simulink model "nonlinsim"  (R2020a)
settings: Solver=VariableStepAuto  StartTime=0.0  StopTime=10.0  RelTol=1e-3
values from neighbouring files (symbols this model uses):
  g = p(6)    [NLS_Dynamics.m]    (also in Project_Problem3.m = 3.711; linsim_script.m = 3.711; nonlinsim_script.m = 3.711)
  Gain = 93298    [linsim_script.m]    (also in nonlinsim_script.m)
  Kd = 9000    [Project_Problem5.m]    (also in linsim_script.m; nonlinsim_script.m = 60000)
  Ki = 1    [Project_Problem5.m]    (also in linsim_script.m = 0.5; nonlinsim_script.m = 200)
  Kp = 5000    [Project_Problem5.m]    (also in linsim_script.m; nonlinsim_script.m = 30000)
  M = p(1)    [NLS_Dynamics.m]    (also in Project_Problem3.m = 1025; linsim_script.m = 1025; nonlinsim_script.m = 1025)
  m = p(2)    [NLS_Dynamics.m]    (also in Project_Problem3.m = 500; linsim_script.m = 500; nonlinsim_script.m = 500)
  Poles = [-0.0008+1.0000i -0.0008-1.0000i -10.23]    [linsim_script.m]    (also in nonlinsim_script.m)
  r1o = 0    [nonlinsim_script.m]
  r2o = 0    [nonlinsim_script.m]
  u1o = (M+m)*g    (= 5659.275)    [nonlinsim_script.m]
  u2o = 0    [nonlinsim_script.m]
  u3o = 0    [nonlinsim_script.m]
  Zeros = [-0.3126 -0.5807 -0.8273]    [linsim_script.m]    (also in nonlinsim_script.m)
libraries: simulink x3
settings Model: Creator=zuzan  LastModifiedBy=zuzan

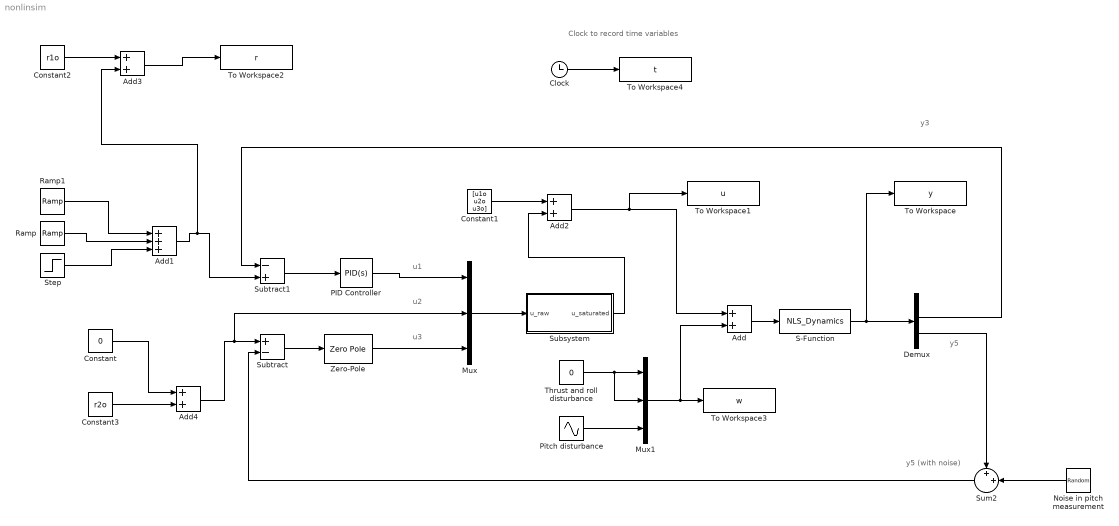
== system nonlinsim ==
  note: y5
  note: u1
  note: y5 (with noise)
  note: u2
  note: Clock to record time variables
  note: y3
  note: u3
  Add{,2..4} (4 alike) : Sum
  Add1 : Sum  Inputs=+++
  Clock : Clock
  Constant : Constant  Value=0
  Constant1 : Constant  Value=[u1o u2o u3o]
  Constant2 : Constant  Value=r1o
  Constant3 : Constant  Value=r2o
  Demux : Demux  Outputs=6
  Mux : Mux  Inputs=3
  Mux1 : Mux  Inputs=3
  Noise in pitch measurement : RandomNumber  Variance=1e-3  SampleTime=0.01
  PID Controller : simulink/Continuous/PID Controller  Controller=PID  Form=Parallel  TimeDomain=Continuous-time  UseExternalTs=off  SampleTime=-1  IntegratorMethod=Forward Euler  FilterMethod=Forward Euler  ControllerParametersSource=internal  P=Kp  I=Ki  D=Kd  UseFilter=on  N=100  TunerSelectOption=Transfer Function Based (PID Tuner App)  InitialConditionSource=internal  InitialConditionForIntegrator=0  InitialConditionForFilter=0  DifferentiatorICPrevScaledInput=0  ExternalReset=none  TrackingMode=off  Kt=1  LimitOutput=off  UpperSaturationLimit=inf  LowerSaturationLimit=-inf  LinearizeAsGain=on  AntiWindupMode=none  Kb=1  POutMin=[]  POutMax=[]  IOutMin=[]  IOutMax=[]  DOutMin=[]  DOutMax=[]  NOutMin=[]  NOutMax=[]  SumOutMin=[]  SumOutMax=[]  SaturationOutMin=[]  SaturationOutMax=[]  PParamMin=[]  PParamMax=[]  IParamMin=[]  IParamMax=[]  DParamMin=[]  DParamMax=[]  NParamMin=[]  NParamMax=[]  KbParamMin=[]  KbParamMax=[]  KtParamMin=[]  KtParamMax=[]  KbOutMin=[]  KbOutMax=[]  KtOutMin=[]  KtOutMax=[]  IntegratorOutMin=[]  IntegratorOutMax=[]  FilterOutMin=[]  FilterOutMax=[]  SumI1OutMin=[]  SumI1OutMax=[]  SumI2OutMin=[]  SumI2OutMax=[]  SumI3OutMin=[]  SumI3OutMax=[]  SumI4OutMin=[]  SumI4OutMax=[]  SumDOutMin=[]  SumDOutMax=[]  DifferentiatorOutMin=[]  DifferentiatorOutMax=[]  FilterDiffOutCoefMin=[]  FilterDiffOutCoefMax=[]  ReciprocalOutMin=[]  ReciprocalOutMax=[]  SumDenOutMin=[]  SumDenOutMax=[]  SumNumOutMin=[]  SumNumOutMax=[]  DivideOutMin=[]  DivideOutMax=[]  UdiffTsProdOutMin=[]  UdiffTsProdOutMax=[]  NTsProdOutMin=[]  NTsProdOutMax=[]  UintegralTsProdOutMin=[]  UintegralTsProdOutMax=[]  UngainTsProdOutMin=[]  UngainTsProdOutMax=[]  IntegratorContinuousStateAttributes=''  IntegratorStateMustResolveToSignalObject=off  IntegratorRTWStateStorageClass=Auto  FilterContinuousStateAttributes=''  FilterStateMustResolveToSignalObject=off  FilterRTWStateStorageClass=Auto  ParallelPVariant=InternalParameters  IdealPVariant=Disabled  IVariant=InternalParameters  DVariant=InternalParameters  IntegratorVariant=Continuous  SatVariant=Disabled  AWVariant=Passthrough  PCopyVariant=Disabled  TRVariant=Disabled  FdbkBlocksVariant=Forward  IdealPFdbkVariant=Disabled  SatFdbkVariant=Disabled  DerivativeFilterVariant=ContFilter  NVariant=InternalParameters  NCopyVariant=Disabled  FilterICVariant=InternalICsFilter  IntegratorICVariant=InternalICs  ExternalResetVariant=Disabled  TRSumVariant=Passthrough  SumFdbkVariant=Disabled  SumVariant=Sum_PID  TsampFilterVariant=InternalTs  TsampNgainVariant=Passthrough  TsampIntegralVariant=Passthrough
  Pitch disturbance : Sin  Amplitude=1e3  SampleTime=0
  Ramp : simulink/Sources/Ramp  slope=0.5  start=0  InitialOutput=0
  Ramp1 : simulink/Sources/Ramp  slope=-0.5  start=40  InitialOutput=0
  S-Function : S-Function  FunctionName=NLS_Dynamics  Parameters=p  SFunctionDeploymentMode=off  EnableBusSupport=off
  Step : Step  Time=40  After=-10  SampleTime=0
  Subsystem : Subsystem
  Subtract : Sum  Inputs=+-
  Subtract1 : Sum  Inputs=-+
  Sum2 : Sum  Inputs=++|
  Thrust and roll disturbance : Constant  Value=0
  To Workspace : ToWorkspace  VariableName=y  SampleTime=-1
  To Workspace1 : ToWorkspace  VariableName=u  SampleTime=-1
  To Workspace2 : ToWorkspace  VariableName=r  SaveFormat=Timeseries  SampleTime=-1
  To Workspace3 : ToWorkspace  VariableName=w  SaveFormat=Timeseries  SampleTime=-1
  To Workspace4 : ToWorkspace  VariableName=t  SampleTime=-1
  Zero-Pole : ZeroPole  Zeros=Zeros  Poles=Poles  Gain=Gain
  wires:
  Sum2/1 -> Subtract/2
  Ramp1/1 -> Add1/1
  Subtract1/1 -> PID Controller/1
  Subtract/1 -> Zero-Pole/1
  Add1/1 -> Add3/2, Subtract1/2
  Subsystem/1(u_saturated) -> Add2/2
  S-Function/1 -> To Workspace/1, Demux/1
  Zero-Pole/1 -> Mux/3
  Add/1 -> S-Function/1
  Thrust and roll disturbance/1 -> Mux1/2, Mux1/1
  Demux/3 -> Subtract1/1
  Ramp/1 -> Add1/2
  Step/1 -> Add1/3
  Mux1/1 -> To Workspace3/1, Add/2
  PID Controller/1 -> Mux/1
  Noise in pitch measurement/1 -> Sum2/2
  Pitch disturbance/1 -> Mux1/3
  Demux/5 -> Sum2/1
  Clock/1 -> To Workspace4/1
  Constant1/1 -> Add2/1
  Mux/1 -> Subsystem/1(u_raw)
  Add2/1 -> Add/1, To Workspace1/1
  Constant2/1 -> Add3/1
  Add3/1 -> To Workspace2/1
  Constant3/1 -> Add4/2
  Constant/1 -> Add4/1
  Add4/1 -> Mux/2, Subtract/1

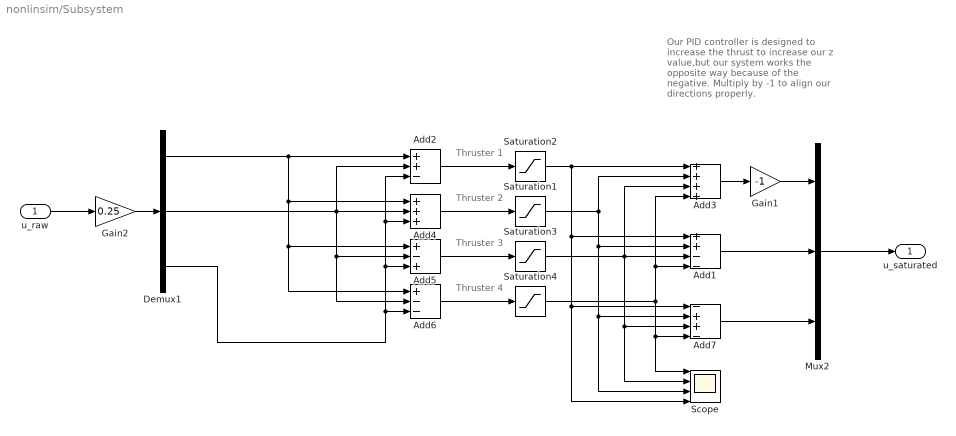
== system nonlinsim/Subsystem ==
  note: Thruster 1
  note: Our PID controller is designed to increase the thrust to increase our z value,but our system works the opposite way because of the negative. Multiply by -1 to align our directions properly.
  note: Thruster 2
  note: Thruster 3
  note: Thruster 4
  u_raw : Inport
  Add1 : Sum  Inputs=++--
  Add2 : Sum  Inputs=++-
  Add3 : Sum  Inputs=++++
  Add4 : Sum  Inputs=+++
  Add5 : Sum  Inputs=+-+
  Add6 : Sum  Inputs=+--
  Add7 : Sum  Inputs=-++-
  Demux1 : Demux  Outputs=3
  Gain1 : Gain  Gain=-1
  Gain2 : Gain  Gain=0.25
  Mux2 : Mux  Inputs=3
  Saturation{1..4} (4 alike) : Saturate  UpperLimit=(M+m)*g  LowerLimit=-(M+m)*g/4
  Scope : Scope  NumInputPorts=4
  u_saturated : Outport
  wires:
  Add6/1 -> Saturation4/1
  Gain2/1 -> Demux1/1
  Saturation3/1 -> Scope/2, Add7/3, Add1/3, Add3/3
  Demux1/2 -> Add2/2, Add5/2, Add6/2, Add4/2
  Add1/1 -> Mux2/2
  Add4/1 -> Saturation1/1
  Saturation4/1 -> Scope/1, Add7/4, Add1/4, Add3/4
  Demux1/3 -> Add2/3, Add4/3, Add5/3, Add6/3
  Add2/1 -> Saturation2/1
  Saturation1/1 -> Scope/3, Add7/2, Add1/2, Add3/2
  u_raw/1 -> Gain2/1
  Add5/1 -> Saturation3/1
  Add7/1 -> Mux2/3
  Mux2/1 -> u_saturated/1
  Demux1/1 -> Add2/1, Add4/1, Add5/1, Add6/1
  Add3/1 -> Gain1/1
  Saturation2/1 -> Add3/1, Scope/4, Add7/1, Add1/1
  Gain1/1 -> Mux2/1
